simulink model "simpSimuRoboToGoKalman"  (R2019b)
settings: Solver=FixedStepDiscrete  StartTime=0.0  StopTime=150.0  FixedStep=0.1  RelTol=1e-3  EnableMultiTasking=on
undefined symbols (not defined in the file): Discrete, Time
libraries: simulink x2, simulink_extras x2, fahrradDiskr x1, ctrlSharedLib x1
settings Model: Creator=pic  LastModifiedBy=mackst
settings SolverCC: ZeroCrossAlgorithm=Adaptive
settings DataIOCC: SaveFormat=Array  TimeSaveName=t  OutputSaveName=y
settings OptimizationCC: ExpressionDepthLimit=2147483647  LifeSpan=inf
settings DebuggingCC: UnderspecifiedInitializationDetection=Classic  MergeDetectMultiDrivingBlocksExec=none  SolverPrmCheckMsg=warning  AllowSymbolicDim=off  StateNameClashWarn=warning  SFUnexpectedBacktrackingDiag=warning  SFNoUnconditionalDefaultTransitionDiag=warning  SFExecutionAtInitializationDiag=none  ArithmeticOperatorsInVariantConditions=warning
settings HardwareCC: ProdBitPerPointer=32  ProdBitPerSizeT=32  ProdBitPerPtrDiffT=32  ProdLargestAtomicFloat=None  ProdIntDivRoundTo=Undefined  ProdEndianess=Unspecified  ProdWordSize=32  ProdHWDeviceType=32-bit Generic
settings ModelReferenceCC: PropagateSignalLabelsOutOfModel=off
settings SFSimCC: SimUseLocalCustomCode=off  CustomCodeUndefinedFunction=UseInterfaceOnly
settings RTWCC: RTWUseLocalCustomCode=off
settings CodeAppCC: StateflowObjectComments=on
settings GRTTargetCC: TargetLangStandard=C89/C90 (ANSI)  CombineOutputUpdateFcns=off  GRTInterface=on
settings ConfigComp: CovMetricSettings=dw  CovSaveCumulativeToWorkspaceVar=on  CovSaveSingleToWorkspaceVar=on  CovExternalEMLEnable=off

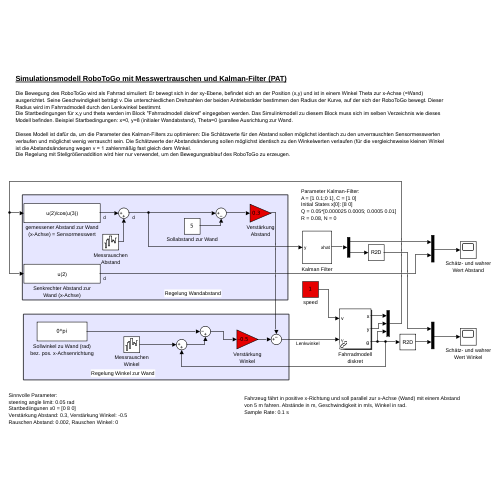
[thumbnail: Simulink's stored preview of the top-level diagram]
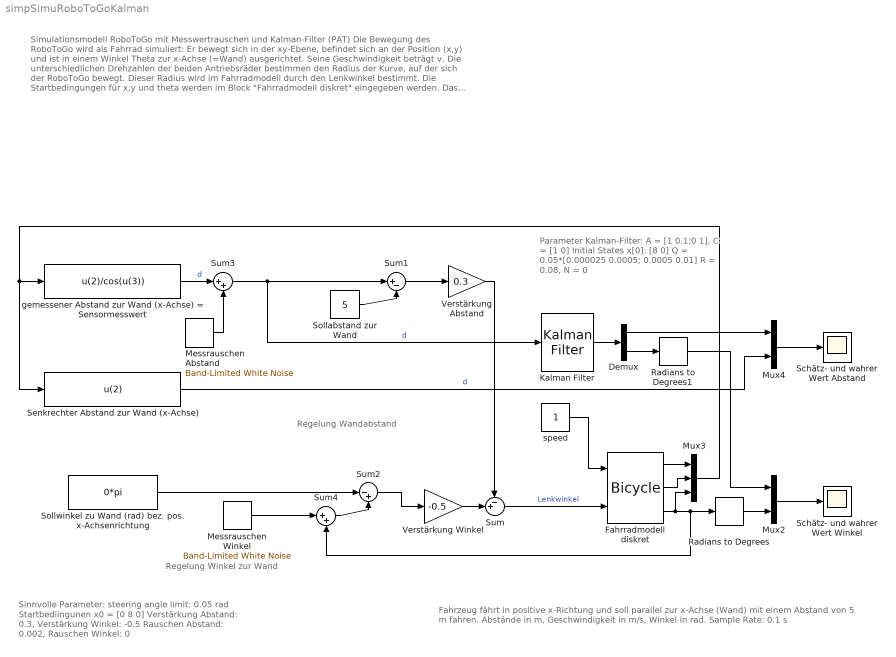
== system simpSimuRoboToGoKalman ==
  note: Sinnvolle Parameter:
      | steering angle limit: 0.05 rad
      | Startbediingunen x0 = [0 8 0]
      | Verstärkung Abstand: 0.3, Verstärkung Winkel: -0.5
      | Rauschen Abstand: 0.002, Rauschen Winkel: 0
  note: Regelung Wandabstand
  note: Regelung Winkel zur Wand
  note: Simulationsmodell RoboToGo mit Messwertrauschen und Kalman-Filter (PAT)
      |
      | Die Bewegung des RoboToGo wird als Fahrrad simuliert: Er bewegt sich in der xy-Ebene, befindet sich an der Position (x,y) und ist in einem Winkel Theta zur x-Achse (=Wand) ausgerichtet. Seine Geschwindigkeit beträgt v. Die unterschiedlichen Drehzahlen der beiden Antriebsräder bestimmen den Radius der Kurve, auf der sich der RoboToGo bewegt. Dieser Radius wird im Fahrradmodell durch den Lenkwinkel bestimmt.
      | Die Startbedingungen für x,y und theta werden im Block "Fahrradmodell diskret" eingegeben werden. Das Simulinkmodell zu diesem Block muss sich im selben Verzeichnis wie dieses Modell befinden. Beispiel Startbedingungen: x=0, y=8 (initialer Wandabstand), Theta=0 (parallee Ausrichtung zur Wand.
      |
      | Dieses Modell ist dafür da, um die Parameter des Kalman-Filters zu optimieren: Die Schätzwerte für den Abstand sollen möglichst identisch zu den unverrauschten Sensormesswerten
      | verlaufen und möglichst wenig verrauscht sein. Die Schätzwerte der Abstandsänderung sollen möglichst identisch zu den Winkelwerten verlaufen (für die vergleichsweise kleinen Winkel
      | ist die Abstandsänderung wegen v = 1 zahlenmäßig fast gleich dem Winkel.
      | Die Regelung mit Stellgrößenaddition wird hier nur verwendet, um den Bewegungsablauf des RoboToGo zu erzeugen.
      |
      | S. Mack, 7.11.2022
  note: Fahrzeug fährt in positive x-Richtung und soll parallel zur x-Achse (Wand) mit einem Abstand
      | von 5 m fahren. Abstände in m, Geschwindigkeit in m/s, Winkel in rad.
      | Sample Rate: 0.1 s
  note: Parameter Kalman-Filter:
      | A = [1 0.1;0 1], C = [1 0]
      | Initial States x[0]: [8 0]
      | Q = 0.05*[0.000025 0.0005; 0.0005 0.01]
      | R = 0.08, N = 0
  Demux : Demux  Outputs=2
  Fahrradmodell diskret : fahrradDiskr/Vehicles/Bicycle  vlim=1  accel=Inf  alim=0.05  steer_rate=Inf  L=1  x0=[0, 8, 0]
  Kalman Filter : ctrlSharedLib/Kalman Filter  TimeDomain=Discrete-Time  UseCurrentEstimator=on  ModelSource=Individual A, B, C, D matrices  ModelSourceVariable=ss(0.95,1,1,0,1)  A=[1 0.1;0 1]  B=0  C=[1 0]  D=0  NumberOfStates=1  NumberOfInputs=1  NumberOfOutputs=1  InitialEstimateSource=Dialog  X0=[8 0]  P0=10  UseK=off  UseGH=off  NumberOfProcessNoiseInputs=1  G=1  TimeInvariantG=on  H=0  TimeInvariantH=on  Q=0.05*[0.000025 0.0005; 0.0005 0.01]  TimeInvariantQ=on  R=0.08  TimeInvariantR=on  N=0  TimeInvariantN=on  AddInputPort=off  AddEnablePort=off  OutputEstimatedY=off  OutputP=off  Ts=0.1
  Messrauschen Abstand : simulink/Sources/Band-Limited White Noise  Cov=[0.002]  Ts=0.1  seed=[23341]
  Messrauschen Winkel : simulink/Sources/Band-Limited White Noise  Cov=[0.001]  Ts=0.1  seed=[23341]
  Mux2 : Mux  Inputs=2
  Mux3 : Mux  Inputs=3
  Mux4 : Mux  Inputs=2
  Radians to Degrees : simulink_extras/Transformations/Radians to Degrees
  Radians to Degrees1 : simulink_extras/Transformations/Radians to Degrees
  Schätz- und wahrer Wert Abstand : Scope
  Schätz- und wahrer Wert Winkel : Scope
  Senkrechter Abstand zur Wand (x-Achse) : Fcn  Expr=u(2)
  Sollabstand zur Wand : Constant  Value=5
  Sollwinkel zu Wand (rad) bez. pos. x-Achsenrichtung : Constant  Value=0*pi
  Sum : Sum  Inputs=-+|
  Sum1 : Sum  Inputs=|+-
  Sum2 : Sum  Inputs=|-+
  Sum3 : Sum  Inputs=|++
  Sum4 : Sum  Inputs=|++
  Verstärkung Abstand : Gain  Gain=0.3
  Verstärkung Winkel : Gain  Gain=-0.5
  gemessener Abstand zur Wand (x-Achse) = Sensormesswert : Fcn  Expr=u(2)/cos(u(3))
  speed : Constant  VectorParams1D=off  SampleTime=-1
  wires:
  Mux3/1 -> Senkrechter Abstand zur Wand (x-Achse)/1, gemessener Abstand zur Wand (x-Achse) = Sensormesswert/1
  Verstärkung Winkel/1 -> Sum/2
  speed/1 -> Fahrradmodell diskret/1
  Sum/1 -> Fahrradmodell diskret/2  "Lenkwinkel"
  Fahrradmodell diskret/1 -> Mux3/1
  Fahrradmodell diskret/2 -> Mux3/2
  Fahrradmodell diskret/3 -> Radians to Degrees/1, Sum4/2, Mux3/3
  Verstärkung Abstand/1 -> Sum/1
  Sum1/1 -> Verstärkung Abstand/1
  Sollabstand zur Wand/1 -> Sum1/2
  Sum3/1 -> Kalman Filter/1, Sum1/1  "d"
  Senkrechter Abstand zur Wand (x-Achse)/1 -> Mux4/2  "d"
  Sum2/1 -> Verstärkung Winkel/1
  Messrauschen Abstand/1 -> Sum3/2
  gemessener Abstand zur Wand (x-Achse) = Sensormesswert/1 -> Sum3/1  "d"
  Messrauschen Winkel/1 -> Sum4/1
  Sollwinkel zu Wand (rad) bez. pos. x-Achsenrichtung/1 -> Sum2/1
  Sum4/1 -> Sum2/2
  Kalman Filter/1 -> Demux/1
  Demux/2 -> Radians to Degrees1/1
  Mux2/1 -> Schätz- und wahrer Wert Winkel/1
  Mux4/1 -> Schätz- und wahrer Wert Abstand/1
  Demux/1 -> Mux4/1
  Radians to Degrees/1 -> Mux2/2
  Radians to Degrees1/1 -> Mux2/1
